simulink model "s4eig"  (Simulink 2.00)
settings: Solver=ode45  StartTime=0.0  StopTime=999999  MaxStep=10  RelTol=1e-3  AbsTol=1e-6
values from neighbouring files (symbols this model uses):
  Domega = 0    [P1HP.M]    (also in PSPH.M)
  H = J*wbm*wbm/(2*Sb)    (= 2.36870505626)    [P1HP.M]    (also in PSPH.M = 1.39074103839)
  Psidso = 0    [M1.M]    (also in M4.M; M4STP.M; M5.M)
  Psipdro = 0    [M1.M]    (also in M4.M; M4STP.M; M5.M; M6.M)
  Psipqro = 0    [M1.M]    (also in M4.M = Vm; M4STP.M = Vm; M5.M; M6.M)
  Psiqso = 0    [M1.M]    (also in M4.M = Vm; M4STP.M = Vm; M5.M; M6.M)
  rpr = 1.99    [P1HP.M]    (also in PSPH.M = 4.12)
  rs = 3.35    [P1HP.M]
  Tfactor = (3*P)/(4*wb)    (= 0.00795774715459)    [P1HP.M]    (also in PSPH.M = 0.00530516476973)
  wb = 2*pi*frated    (= 376.991118431)    [P1HP.M]    (also in PSPH.M)
  we = wb    (= 376.991118431)    [P1HP.M]    (also in PSPH.M)
  wrbywbo = 0    [M1.M]    (also in M4.M = 1; M4STP.M = 1; M5.M; M6.M)
  xls = 6.94e-3*wb    (= 2.61631836191)    [P1HP.M]
  xM = 1/(1/xm + 1/xls + 1/xplr)    (= 1.2810101836)    [P1HP.M]
  xplr = xls    (= 2.61631836191)    [P1HP.M]    (also in PSPH.M = 2.12)
settings Model: SaveTime=off  SaveOutput=off  ConsistencyChecking=off

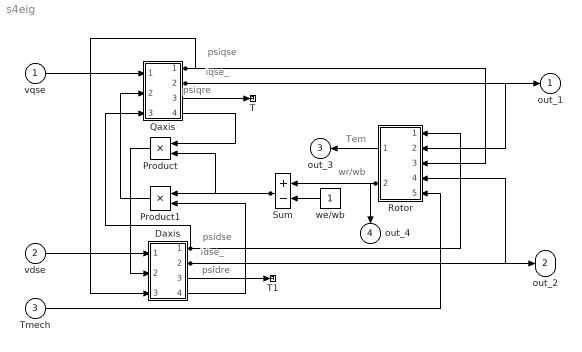
== system s4eig ==
  note: psiqre
  note: psidse
  note: idse_
  note: psiqse
  note: iqse_
  note: psidre
  note: Tem
  note: wr/wb
  vqse : Inport  Port=1  PortWidth=-1  SampleTime=-1
  vdse : Inport  Port=2  PortWidth=-1  SampleTime=-1
  Tmech : Inport  Port=3  PortWidth=-1  SampleTime=-1
  Daxis : Subsystem
  Product : Product  Orientation=left  Inputs=2
  Product1 : Product  Orientation=left  Inputs=2
  Qaxis : Subsystem
  Rotor : Subsystem  Orientation=left
  Sum : Sum  Orientation=left  Inputs=+-
  T : Terminator
  T1 : Terminator
  we/wb : Constant  Orientation=left  Value=1
  out_1 : Outport  Port=1  InitialOutput=0
  out_2 : Outport  Port=2  InitialOutput=0
  out_3 : Outport  Orientation=left  Port=3  InitialOutput=0
  out_4 : Outport  Orientation=down  Port=4  InitialOutput=0
  wires:
  Sum/1 -> Product1/1, Product/2
  we/wb/1 -> Sum/2
  Product1/1 -> Qaxis/2((wr-we)*psidr'/wb)
  Product/1 -> Daxis/2(in_(wr/wb)*psiqr')
  Daxis/1(out_psids) -> Qaxis/3(in_psids), Rotor/1(in_psidse)
  Qaxis/4(out_psiqr') -> Product/1
  vqse/1 -> Qaxis/1(in_vqs)
  Qaxis/2(out_iqs) -> Rotor/2(in_iqse), out_1/1
  Rotor/1(out_Tem) -> out_3/1
  Rotor/2(out_wr/wb) -> Sum/1, out_4/1
  Tmech/1 -> Rotor/5(in_Tmech)
  vdse/1 -> Daxis/1(in_vds)
  Daxis/2(out_ids) -> Rotor/4(in_idse), out_2/1
  Qaxis/1(out_psiqs) -> Rotor/3(in_psiqse), Daxis/3(in_psiqs)
  Daxis/4(out_psidr') -> Product1/2
  Qaxis/3(out_iqr') -> T/1
  Daxis/3(out_idr') -> T1/1

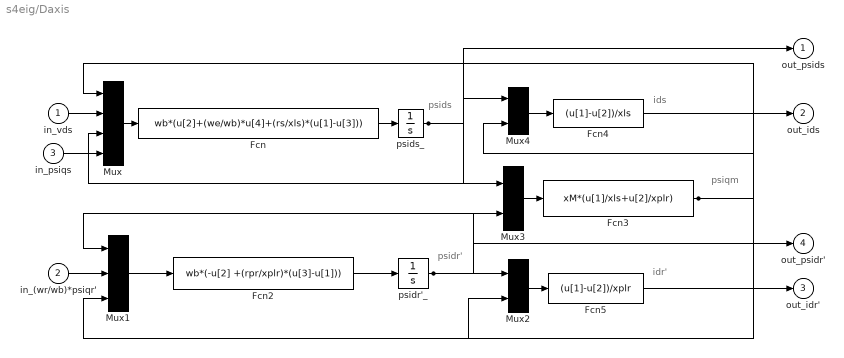
== system s4eig/Daxis ==
  note: psidr'
  note: idr'
  note: psiqm
  note: psids
  note: ids
  in_vds : Inport  Port=1  PortWidth=-1  SampleTime=-1
  in_(wr/wb)*psiqr' : Inport  Port=2  PortWidth=-1  SampleTime=-1
  in_psiqs : Inport  Port=3  PortWidth=-1  SampleTime=-1
  Fcn : Fcn  Expr=wb*(u[2]+(we/wb)*u[4]+(rs/xls)*(u[1]-u[3]))
  Fcn2 : Fcn  Expr=wb*(-u[2] +(rpr/xplr)*(u[3]-u[1]))
  Fcn3 : Fcn  Expr=xM*(u[1]/xls+u[2]/xplr)
  Fcn4 : Fcn  Expr=(u[1]-u[2])/xls
  Fcn5 : Fcn  Expr=(u[1]-u[2])/xplr
  Mux : Mux  Inputs=4
  Mux1 : Mux  Inputs=3
  Mux2 : Mux  Inputs=2
  Mux3 : Mux  Inputs=2
  Mux4 : Mux  Inputs=2
  psidr'_ : Integrator  ExternalReset=none  InitialConditionSource=internal  InitialCondition=Psipdro  LimitOutput=off  UpperSaturationLimit=inf  LowerSaturationLimit=-inf  ShowSaturationPort=off  ShowStatePort=off  AbsoluteTolerance=auto
  psids_ : Integrator  ExternalReset=none  InitialConditionSource=internal  InitialCondition=Psidso  LimitOutput=off  UpperSaturationLimit=inf  LowerSaturationLimit=-inf  ShowSaturationPort=off  ShowStatePort=off  AbsoluteTolerance=auto
  out_psids : Outport  Port=1  InitialOutput=0
  out_ids : Outport  Port=2  InitialOutput=0
  out_idr' : Outport  Port=3  InitialOutput=0
  out_psidr' : Outport  Port=4  InitialOutput=0
  wires:
  Mux2/1 -> Fcn5/1
  psidr'_/1 -> Mux2/1, Mux3/2, Mux1/1, out_psidr'/1
  Mux1/1 -> Fcn2/1
  Fcn3/1 -> Mux2/2, Mux/1, Mux1/3, Mux4/2
  psids_/1 -> Mux/3, Mux4/1, Mux3/1, out_psids/1
  Mux4/1 -> Fcn4/1
  Mux3/1 -> Fcn3/1
  Fcn2/1 -> psidr'_/1
  Fcn/1 -> psids_/1
  Mux/1 -> Fcn/1
  Fcn4/1 -> out_ids/1
  in_vds/1 -> Mux/2
  in_(wr/wb)*psiqr'/1 -> Mux1/2
  Fcn5/1 -> out_idr'/1
  in_psiqs/1 -> Mux/4

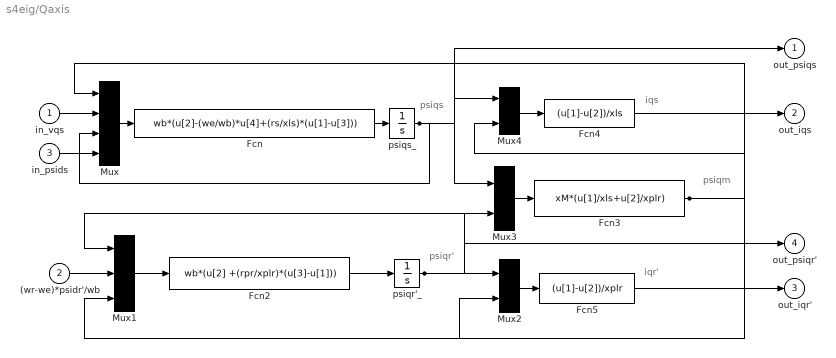
== system s4eig/Qaxis ==
  note: psiqr'
  note: iqr'
  note: psiqm
  note: psiqs
  note: iqs
  in_vqs : Inport  Port=1  PortWidth=-1  SampleTime=-1
  (wr-we)*psidr'/wb : Inport  Port=2  PortWidth=-1  SampleTime=-1
  in_psids : Inport  Port=3  PortWidth=-1  SampleTime=-1
  Fcn : Fcn  Expr=wb*(u[2]-(we/wb)*u[4]+(rs/xls)*(u[1]-u[3]))
  Fcn2 : Fcn  Expr=wb*(u[2] +(rpr/xplr)*(u[3]-u[1]))
  Fcn3 : Fcn  Expr=xM*(u[1]/xls+u[2]/xplr)
  Fcn4 : Fcn  Expr=(u[1]-u[2])/xls
  Fcn5 : Fcn  Expr=(u[1]-u[2])/xplr
  Mux : Mux  Inputs=4
  Mux1 : Mux  Inputs=3
  Mux2 : Mux  Inputs=2
  Mux3 : Mux  Inputs=2
  Mux4 : Mux  Inputs=2
  psiqr'_ : Integrator  ExternalReset=none  InitialConditionSource=internal  InitialCondition=Psipqro  LimitOutput=off  UpperSaturationLimit=inf  LowerSaturationLimit=-inf  ShowSaturationPort=off  ShowStatePort=off  AbsoluteTolerance=auto
  psiqs_ : Integrator  ExternalReset=none  InitialConditionSource=internal  InitialCondition=Psiqso  LimitOutput=off  UpperSaturationLimit=inf  LowerSaturationLimit=-inf  ShowSaturationPort=off  ShowStatePort=off  AbsoluteTolerance=auto
  out_psiqs : Outport  Port=1  InitialOutput=0
  out_iqs : Outport  Port=2  InitialOutput=0
  out_iqr' : Outport  Port=3  InitialOutput=0
  out_psiqr' : Outport  Port=4  InitialOutput=0
  wires:
  Mux2/1 -> Fcn5/1
  psiqr'_/1 -> Mux2/1, Mux3/2, Mux1/1, out_psiqr'/1
  Mux1/1 -> Fcn2/1
  Fcn3/1 -> Mux2/2, Mux/1, Mux1/3, Mux4/2
  psiqs_/1 -> Mux/3, Mux4/1, Mux3/1, out_psiqs/1
  Mux4/1 -> Fcn4/1
  Mux3/1 -> Fcn3/1
  Fcn2/1 -> psiqr'_/1
  Fcn/1 -> psiqs_/1
  Mux/1 -> Fcn/1
  Fcn4/1 -> out_iqs/1
  in_vqs/1 -> Mux/2
  (wr-we)*psidr'/wb/1 -> Mux1/2
  Fcn5/1 -> out_iqr'/1
  in_psids/1 -> Mux/4

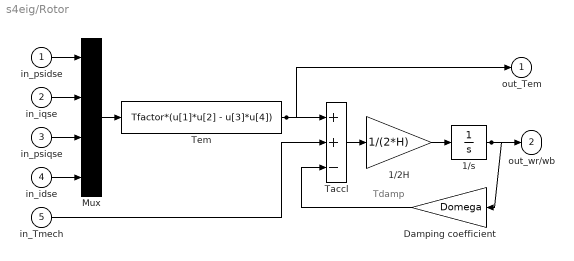
== system s4eig/Rotor ==
  note: Tdamp
  in_psidse : Inport  Port=1  PortWidth=-1  SampleTime=-1
  in_iqse : Inport  Port=2  PortWidth=-1  SampleTime=-1
  in_psiqse : Inport  Port=3  PortWidth=-1  SampleTime=-1
  in_idse : Inport  Port=4  PortWidth=-1  SampleTime=-1
  in_Tmech : Inport  Port=5  PortWidth=-1  SampleTime=-1
  1/2H : Gain  Gain=1/(2*H)
  1/s : Integrator  ExternalReset=none  InitialConditionSource=internal  InitialCondition=wrbywbo  LimitOutput=off  UpperSaturationLimit=inf  LowerSaturationLimit=-inf  ShowSaturationPort=off  ShowStatePort=off  AbsoluteTolerance=auto
  Damping coefficient : Gain  Orientation=left  Gain=Domega
  Mux : Mux  Inputs=4
  Taccl : Sum  Inputs=++-
  Tem : Fcn  Expr=Tfactor*(u[1]*u[2] - u[3]*u[4])
  out_Tem : Outport  Port=1  InitialOutput=0
  out_wr/wb : Outport  Port=2  InitialOutput=0
  wires:
  Damping coefficient/1 -> Taccl/3
  Tem/1 -> out_Tem/1, Taccl/1
  1/2H/1 -> 1/s/1
  Taccl/1 -> 1/2H/1
  in_Tmech/1 -> Taccl/2
  1/s/1 -> Damping coefficient/1, out_wr/wb/1
  Mux/1 -> Tem/1
  in_psidse/1 -> Mux/1
  in_iqse/1 -> Mux/2
  in_psiqse/1 -> Mux/3
  in_idse/1 -> Mux/4
